simulink model "test_daidalus_sfunc_block"  (R2018b)
settings: Solver=FixedStepDiscrete  StartTime=0.0  StopTime=0  FixedStep=1  RelTol=1e-3  EnableMultiTasking=on
undefined symbols (not defined in the file or in its folder): DEGAS, dh_ftps, e_ft, enuStateEstimate, h_ft, n_ft, phi_rad, psi_rad, theta_rad, v_ftps
libraries: DaidalusV101Block x1, NullAircraftEstimateBus x1, NullAircraftStateBus x1
settings Model: Creator=RA24876  LastModifiedBy=BI28030
settings DataIOCC: LimitDataPoints=on  MaxDataPoints=10000  SaveFormat=StructureWithTime  SignalLogging=off  DSMLogging=off  SaveTime=off  OutputSaveName=youtNew
settings OptimizationCC: LifeSpan=inf
settings DebuggingCC: SFUnexpectedBacktrackingDiag=warning  SFNoUnconditionalDefaultTransitionDiag=warning  SFExecutionAtInitializationDiag=none
settings HardwareCC: ProdBitPerPointer=32  ProdBitPerSizeT=32  ProdBitPerPtrDiffT=32  ProdLargestAtomicFloat=None  ProdIntDivRoundTo=Undefined  ProdEndianess=Unspecified  ProdWordSize=32  ProdHWDeviceType=32-bit Generic
settings ModelReferenceCC: PropagateSignalLabelsOutOfModel=off
settings SFSimCC: SimUseLocalCustomCode=off
settings RTWCC: RTWUseLocalCustomCode=off
settings CodeAppCC: StateflowObjectComments=on
settings GRTTargetCC: TargetLangStandard=C89/C90 (ANSI)  GeneratePreprocessorConditionals=Disable all
settings ConfigComp: CovMetricSettings=dw  CovHtmlReporting=on  CovSaveCumulativeToWorkspaceVar=on  CovSaveSingleToWorkspaceVar=on  CovExternalEMLEnable=off

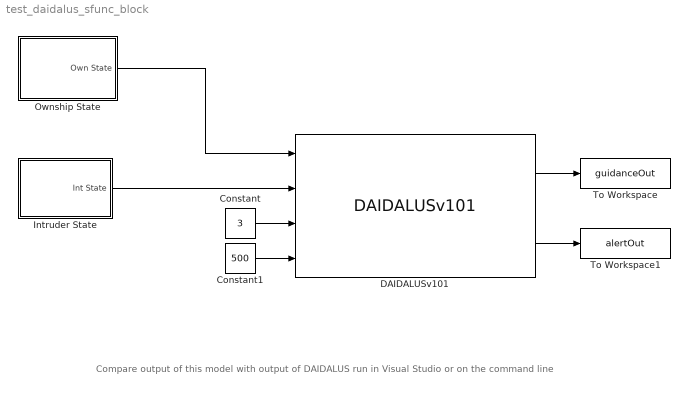
== system test_daidalus_sfunc_block ==
  note: Compare output of this model with output of DAIDALUS run in Visual Studio or on the command line
  Constant : Constant  Value=3
  Constant1 : Constant  Value=500
  DAIDALUSv101 : DaidalusV101Block/DAIDALUSv101  DTHR=daa_guideDTHR  ZTHR=daa_guideZTHR  TTHR=daa_guideTTHR  TCOA=daa_guideTCOA  lookahead_time=daa_guideLookahead  use_single_direction=daa_singleDirRecovery  prev_DTHR=daa_prevDTHR  prev_ZTHR=daa_prevZTHR  prev_TTHR=daa_prevTTHR  prev_TCOA=daa_prevTCOA  prev_lookahead=daa_prevLookahead  prev_early=daa_prevEarly  corr_DTHR=daa_corrDTHR  corr_ZTHR=daa_corrZTHR  corr_TTHR=daa_corrTTHR  corr_TCOA=daa_corrTCOA  corr_lookahead=daa_corrLookahead  corr_early=daa_corrEarly  warn_DTHR=daa_warnDTHR  warn_ZTHR=daa_warnZTHR  warn_TTHR=daa_warnTTHR  warn_TCOA=daa_warnTCOA  warn_lookahead=daa_warnLookahead  warn_early=daa_warnEarly  min_alt=daa_minAlt  rec_stab_time=daa_recStabTime  min_hor_rec=daa_minHorRec  ca_factor=daa_caFactor
  Intruder State : Subsystem  mask{pos_east=0, pos_north=5, pos_up=3000, vel_east=0, vel_north=-100, vel_up=0}
      mask prompts: pos_east "Position East (nmi)"; pos_north "Position North (nmi)"; pos_up "Altitude (ft)"; vel_east "Velocity East (kt)"; vel_north "Velocity North (kt)"; vel_up "Vertical Rate (fpm)"
  Ownship State : Subsystem  mask{pos_east=0, pos_north=0, pos_up=3000, vel_east=0, vel_north=100, vel_up=0}
      mask prompts: pos_east "Position East (nmi)"; pos_north "Position North (nmi)"; pos_up "Altitude (ft)"; vel_east "Velocity East (kt)"; vel_north "Velocity North (kt)"; vel_up "Vertical Rate (fpm)"
  To Workspace : ToWorkspace  VariableName=guidanceOut  SampleTime=-1
  To Workspace1 : ToWorkspace  VariableName=alertOut  SampleTime=-1
  wires:
  Constant/1 -> DAIDALUSv101/3
  Constant1/1 -> DAIDALUSv101/4
  DAIDALUSv101/1 -> To Workspace/1
  DAIDALUSv101/2 -> To Workspace1/1
  Intruder State/1(Int State) -> DAIDALUSv101/2
  Ownship State/1(Own State) -> DAIDALUSv101/1

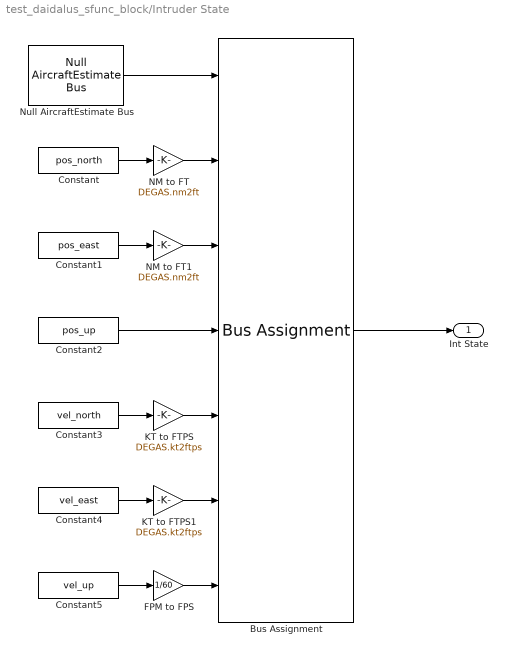
== system test_daidalus_sfunc_block/Intruder State ==
  Bus Assignment : BusAssignment  AssignedSignals=enuStateEstimate.n_ft,enuStateEstimate.e_ft,enuStateEstimate.h_ft,enuStateEstimate.dn_ftps,enuStateEstimate.de_ftps,enuStateEstimate.dh_ftps
  Constant : Constant  Value=pos_north
  Constant1 : Constant  Value=pos_east
  Constant2 : Constant  Value=pos_up
  Constant3 : Constant  Value=vel_north
  Constant4 : Constant  Value=vel_east
  Constant5 : Constant  Value=vel_up
  FPM to FPS : Gain  Gain=1/60
  KT to FTPS : Gain  Gain=DEGAS.kt2ftps
  KT to FTPS1 : Gain  Gain=DEGAS.kt2ftps
  NM to FT : Gain  Gain=DEGAS.nm2ft
  NM to FT1 : Gain  Gain=DEGAS.nm2ft
  Null AircraftEstimate Bus : NullAircraftEstimateBus/Null AircraftEstimate Bus
  Int State : Outport
  wires:
  Null AircraftEstimate Bus/1 -> Bus Assignment/1
  Bus Assignment/1 -> Int State/1
  Constant1/1 -> NM to FT1/1
  Constant2/1 -> Bus Assignment/4
  Constant3/1 -> KT to FTPS/1
  Constant4/1 -> KT to FTPS1/1
  Constant5/1 -> FPM to FPS/1
  Constant/1 -> NM to FT/1
  NM to FT/1 -> Bus Assignment/2
  NM to FT1/1 -> Bus Assignment/3
  KT to FTPS/1 -> Bus Assignment/5
  KT to FTPS1/1 -> Bus Assignment/6
  FPM to FPS/1 -> Bus Assignment/7

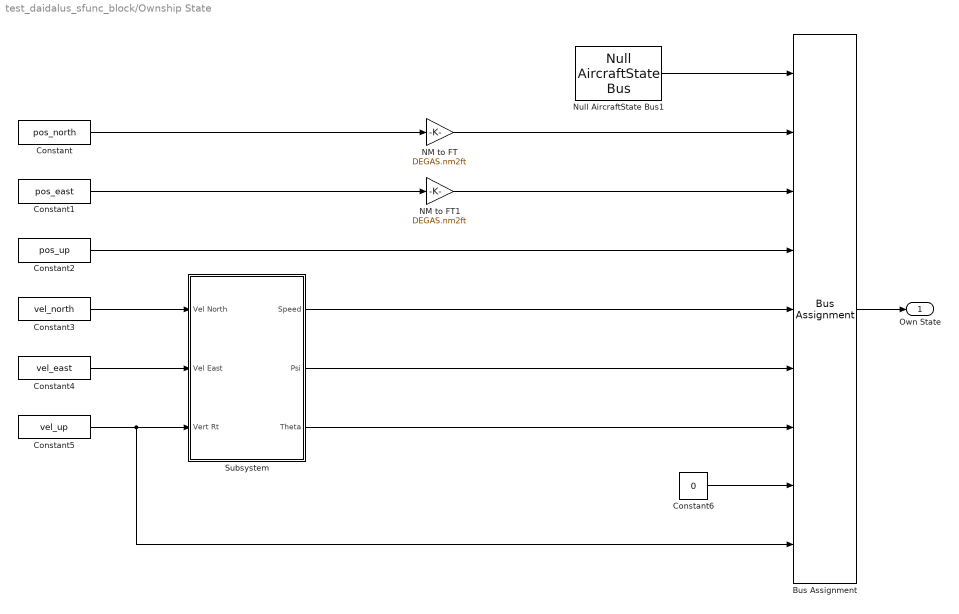
== system test_daidalus_sfunc_block/Ownship State ==
  Bus Assignment : BusAssignment  AssignedSignals=n_ft,e_ft,h_ft,v_ftps,psi_rad,theta_rad,phi_rad,dh_ftps
  Constant : Constant  Value=pos_north
  Constant1 : Constant  Value=pos_east
  Constant2 : Constant  Value=pos_up
  Constant3 : Constant  Value=vel_north
  Constant4 : Constant  Value=vel_east
  Constant5 : Constant  Value=vel_up
  Constant6 : Constant  Value=0
  NM to FT : Gain  Gain=DEGAS.nm2ft
  NM to FT1 : Gain  Gain=DEGAS.nm2ft
  Null AircraftState Bus1 : NullAircraftStateBus/Null AircraftState Bus
  Subsystem : Subsystem
  Own State : Outport
  wires:
  Bus Assignment/1 -> Own State/1
  Null AircraftState Bus1/1 -> Bus Assignment/1
  Constant1/1 -> NM to FT1/1
  Constant/1 -> NM to FT/1
  Constant3/1 -> Subsystem/1(Vel North)
  Constant4/1 -> Subsystem/2(Vel East)
  Constant5/1 -> Bus Assignment/9, Subsystem/3(Vert Rt)
  Subsystem/1(Speed) -> Bus Assignment/5
  Subsystem/2(Psi) -> Bus Assignment/6
  Subsystem/3(Theta) -> Bus Assignment/7
  Constant6/1 -> Bus Assignment/8
  NM to FT/1 -> Bus Assignment/2
  NM to FT1/1 -> Bus Assignment/3
  Constant2/1 -> Bus Assignment/4

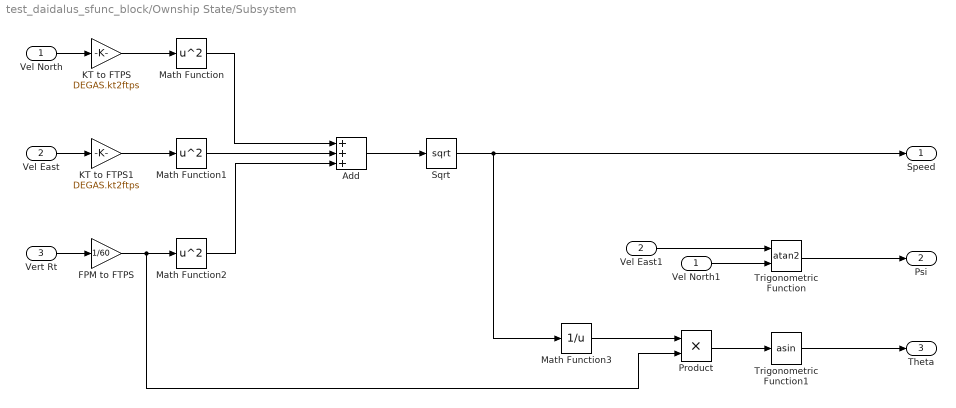
== system test_daidalus_sfunc_block/Ownship State/Subsystem ==
  Vel North : Inport
  Vel East : Inport  Port=2
  Vert Rt : Inport  Port=3
  Add : Sum  Inputs=+++
  FPM to FTPS : Gain  Gain=1/60
  KT to FTPS : Gain  Gain=DEGAS.kt2ftps
  KT to FTPS1 : Gain  Gain=DEGAS.kt2ftps
  Math Function : Math  Operator=square  SaturateOnIntegerOverflow=on
  Math Function1 : Math  Operator=square  SaturateOnIntegerOverflow=on
  Math Function2 : Math  Operator=square  SaturateOnIntegerOverflow=on
  Math Function3 : Math  Operator=reciprocal  SaturateOnIntegerOverflow=on
  Product : Product
  Sqrt : Sqrt  SaturateOnIntegerOverflow=on
  Trigonometric Function : Trigonometry  Operator=atan2
  Trigonometric Function1 : Trigonometry  Operator=asin
  Vel East1 : InportShadow  Port=2
  Vel North1 : InportShadow
  Speed : Outport
  Psi : Outport  Port=2
  Theta : Outport  Port=3
  wires:
  Vel North/1 -> KT to FTPS/1
  Vel East/1 -> KT to FTPS1/1
  Vert Rt/1 -> FPM to FTPS/1
  Math Function/1 -> Add/1
  Math Function1/1 -> Add/2
  Math Function2/1 -> Add/3
  Add/1 -> Sqrt/1
  KT to FTPS/1 -> Math Function/1
  KT to FTPS1/1 -> Math Function1/1
  FPM to FTPS/1 -> Product/2, Math Function2/1
  Sqrt/1 -> Math Function3/1, Speed/1
  Trigonometric Function/1 -> Psi/1
  Vel East1/1 -> Trigonometric Function/1
  Vel North1/1 -> Trigonometric Function/2
  Trigonometric Function1/1 -> Theta/1
  Math Function3/1 -> Product/1
  Product/1 -> Trigonometric Function1/1
